simulink model "Team37_Quadcopter_Simulation"  (R2018a)
settings: Solver=ode45  StartTime=0  StopTime=10.0  FixedStep=0.005  RelTol=1e-3  EnableMultiTasking=on
model workspace (MAT data in the model file):
  Sig = Simulink.Signal
  Sig.DataType = 'auto'
  Sig.Dimensions = -1
  Sig.DimensionsMode = 'auto'
  Sig.Complexity = 'auto'
  Sig.SampleTime = -1
  Sig.SamplingMode = 'auto'
values from neighbouring files (symbols this model uses):
  IC =     [ICload.mat]
undefined symbols (not defined in the file or in its folder): DiscIntNeverNeededParam, quadModel
libraries: simulink x8
(part 1 of 2)
Description:
  | This is a configurable quadcopter simulation.
  | This Simulink model demonstates several effects intended to simulate a real-world attitude control implementation.
  | 
  | Additional quadcopter modeling and simulation materials available at:
  | github.com/dch33/Quad-Sim
  | 
  | Copyright (C) 2014 D. Hartman, K. Landis, S. Moreno, J. Kim, M. Mehrer
  | 
  | License:
  |     This program is free software: you can redistribute it and/or modify
  |     it under the terms of the GNU LESSER GENERAL PUBLIC LICENSE as published by
  |     the Free Software Foundation, either version 3 of the License, or
  |     (at your option) any later version.
  | 
  |     This program is distributed in the hope that it will be useful,
  |     but WITHOUT ANY WARRANTY; without even the implied warranty of
  |     MERCHANTABILITY or FITNESS FOR A PARTICULAR PURPOSE.  See the
  |     GNU General Public License for more details.
  | 
  |     You should have received a copy of the GNU LESSER GENERAL PUBLIC LICENSE
  |     along with this program.  If not, see <http://www.gnu.org/licenses/>.
settings Model: ModifiedComment=m203876 -- Mon Sep 02 20:57:19 2019 -- Version 1.4  Creator=David Hartman  LastModifiedBy=m203876
settings Model: ModifiedHistory=|
  | m203876 -- Mon Sep 02 20:57:19 2019 -- Version 1.4
  | 
  | davidhartman -- Fri Jun 06 23:02:32 2014 -- Version 1.3
settings SolverCC: AutoInsertRateTranBlk=on
settings DataIOCC: SaveFormat=Array  SaveState=on  SignalLogging=off
settings OptimizationCC: DefaultParameterBehavior=Inlined  LifeSpan=inf
settings DebuggingCC: UnderspecifiedInitializationDetection=Classic  MergeDetectMultiDrivingBlocksExec=none  SolverPrmCheckMsg=warning  UniqueDataStoreMsg=warning  StateNameClashWarn=warning  StrictBusMsg=WarnOnBusTreatedAsVector  SFUnexpectedBacktrackingDiag=warning  SFNoUnconditionalDefaultTransitionDiag=warning  SFExecutionAtInitializationDiag=none
settings HardwareCC: ProdBitPerPointer=32  ProdBitPerSizeT=32  ProdBitPerPtrDiffT=32  ProdLargestAtomicFloat=None  ProdIntDivRoundTo=Undefined  ProdEndianess=Unspecified  ProdWordSize=32  ProdHWDeviceType=32-bit Generic
settings ModelReferenceCC: PropagateSignalLabelsOutOfModel=off
settings CodeAppCC: StateflowObjectComments=on
settings GRTTargetCC: TargetLangStandard=C89/C90 (ANSI)  GeneratePreprocessorConditionals=Disable all
settings ConfigComp: CovMetricSettings=dw  CovHtmlReporting=on  CovSaveCumulativeToWorkspaceVar=on  CovSaveSingleToWorkspaceVar=on  CovExternalEMLEnable=off

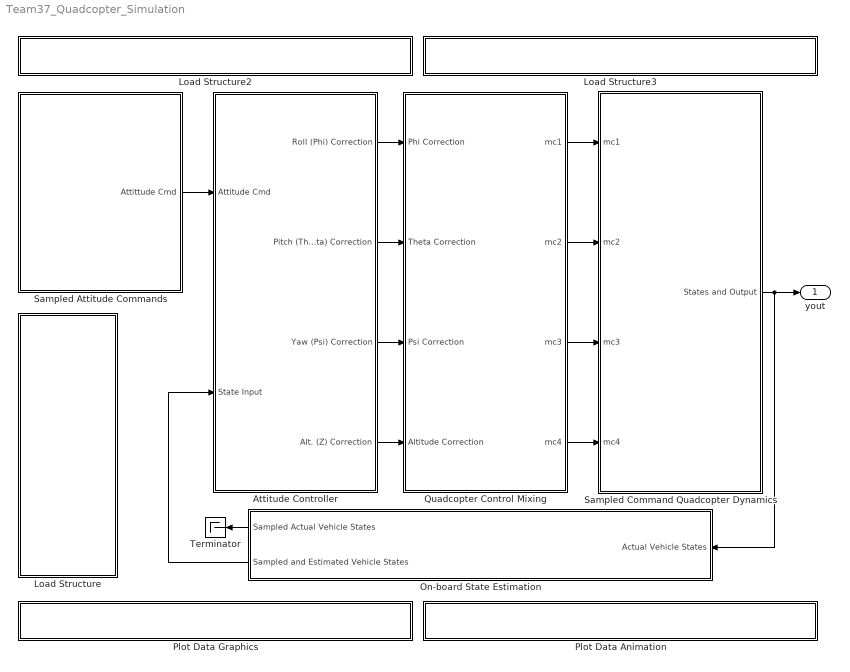
== system Team37_Quadcopter_Simulation ==
  Attitude Controller : Subsystem
  Load Structure : Subsystem
      settings: OpenFcn=|
      | uiopen('load')
      | if (exist('IC')==1 && exist('quadModel')==1)
      | set_param(bdroot, 'SimulationCommand', 'update')
      | end
      mask Display: fprintf('LOAD:\nQuadcopter\nModel Or\nInitial\nConditions');
  Load Structure2 : Subsystem
      settings: OpenFcn=|
      | if exist('GUI_Modeling') == 2,
      | run('GUI_Modeling')
      | 
      | else
      | 
      | msgbox('The desired GUI must be first added to MATLABs path.')
      | 
      | end
      mask Display: fprintf('OPEN GUI: Build New \n Model');
  Load Structure3 : Subsystem
      settings: OpenFcn=|
      | if exist('GUI_IC') == 2,
      | run('GUI_IC')
      | 
      | else
      | 
      | msgbox('The desired GUI must be first added to MATLABs path.')
      | 
      | end
      mask Display: fprintf('OPEN GUI: Create Initial \n Conditions');
  On-board State Estimation : Subsystem  mask{ControllerSampleTime=1/200, Gyro_Alpha=0.50, Accel_Alpha=0.06, EAComp=0.92}
      mask prompts: ControllerSampleTime "State sensor sampling time (s):"; Gyro_Alpha "Gyro Alpha Value:"; Accel_Alpha "Accelerometer Alpha Value:"; EAComp "Complimentary Filter Alpha (must be between 0 and 1):"
      mask Help:
      | Sampling Time: A typical value might be 0.02 to 0.002 seconds (50 Hz to 400 Hz)
      | depending on the control system and sensors used. For best simulink performance,
      | it may be necessarry to round the value a bit to achieve an integer multiple
      | relationship between motor command sampling time and state estimation sampling time.
      | See simulink documentation for more details.
      mask TypeOptions ControllerSampleTime: Rate Transition/OutPortSampleTime
      mask TypeOptions Gyro_Alpha: filterRawData()/Gyro_Alpha
      mask TypeOptions Accel_Alpha: filterRawData()/Accel_Alpha
      mask TypeOptions EAComp: State Estimation and Complimentary Mixing/EAComp
      mask Display:
      | fprintf(['Sampling Time: ' num2str(ControllerSampleTime) ' (s)']);
      | fprintf(['\n \n' num2str(1/ControllerSampleTime) ' Hz']);
  Plot Data Animation : Subsystem
      settings: OpenFcn=|
      | if exist('QuadAnim4') == 2,
      |     if exist('yout')
      | 	run('QuadAnim4');
      |     else
      |     msgbox('Simulation must be run before data can be plotted.');
      |     end
      | else                                                                          msgbox('The desired GUI must be first added to MATLABs path.')
      | end
      mask Display: fprintf('OPEN GUI: Flight Animation')
  Plot Data Graphics : Subsystem
      settings: OpenFcn=|
      | if exist('yout')
      | yout = evalin('base', 'yout');
      | tout = evalin('base', 'tout');
      | quadPlots(yout, tout)
      | else
      | msgbox('Simulation must be run before data can be plotted.')
      | end
      mask Display: fprintf('OPEN PLOT: State Data')
  Quadcopter Control Mixing : Subsystem  mask{QuantizationInterval=0.1}
      mask prompts: QuantizationInterval "Quantization interval (% throttle):"
      mask help:
      | Input desired quantization interval as Percent Throttle.
      | For example, if PWM ESC command signals are restricted to integers between
      | 1000 and 2000 us, quantization would be 0.1 % throttle.
      mask TypeOptions QuantizationInterval:
      | Quantizer1
      | /QuantizationInterval | Quantizer2
      | /QuantizationInterval | Quantizer3
      | /QuantizationInterval | Quantizer4/QuantizationInterval
      mask Display:
      | fprintf(['Quantization : ' num2str(QuantizationInterval) '%%  Throttle']);
      | modelLoaded = evalin('base','exist(''quadModel'',''var'')');
      | if (modelLoaded==1)
      |     if (evalin('base','quadModel.plusConfig'))
      |     fprintf([' \n' ' \n'  'Configuration "+"']);
      |     else if (~evalin('base','quadModel.plusConfig'))
      |         fprintf([' \n' ' \n' 'Configuration "X"']);
      |         end
      |     end
      | else
      |     fprintf([' \n' ' \n'  'Model Not Loaded']);
      | end
  Sampled Attitude Commands : Subsystem  mask{CommandSampleTime=1/200}
      mask prompts: CommandSampleTime "Attitude Command Sample Time (s):"
      mask TypeOptions CommandSampleTime: Rate Transition/OutPortSampleTime
      mask Display:
      | fprintf(['Sampling Time: ' num2str(CommandSampleTime) ' (s)\n\n\n\n\n\n\n']);
      | fprintf(['\n \n' num2str(1/CommandSampleTime) ' Hz \n\n\n\n\n\n']);
  Sampled Command Quadcopter Dynamics : Subsystem  mask{ESCSampleTime=0.02}
      mask prompts: ESCSampleTime "Motor Command Sampling Time (s):"
      mask help:
      | Input sampling rate for motor commands in seconds.
      | This rate will be applied to simulate the propagation of controller commands to the ESC's.
      | A typical value is on the order of 0.02 seconds (50 Hz).
      mask TypeOptions ESCSampleTime: Rate Transition/OutPortSampleTime
      mask Display:
      | fprintf(['Sampling Time: ' num2str(ESCSampleTime) ' (s)\n\n\n\n\n\n']);
      | fprintf(['\n \n' num2str(1/ESCSampleTime) ' Hz\n\n\n\n\n']);
  Terminator : Terminator
  yout : Outport
  wires:
  Sampled Command Quadcopter Dynamics/1(States and Output) -> yout/1, On-board State Estimation/1(Actual Vehicle States)
  Quadcopter Control Mixing/1(mc1) -> Sampled Command Quadcopter Dynamics/1(mc1)
  Quadcopter Control Mixing/2(mc2) -> Sampled Command Quadcopter Dynamics/2(mc2)
  Quadcopter Control Mixing/3(mc3) -> Sampled Command Quadcopter Dynamics/3(mc3)
  Quadcopter Control Mixing/4(mc4) -> Sampled Command Quadcopter Dynamics/4(mc4)
  Attitude Controller/1(Roll (Phi) Correction) -> Quadcopter Control Mixing/1(Phi Correction)
  Attitude Controller/3(Yaw (Psi) Correction) -> Quadcopter Control Mixing/3(Psi Correction)
  Attitude Controller/2(Pitch (Theta) Correction) -> Quadcopter Control Mixing/2(Theta Correction)
  Attitude Controller/4(Alt. (Z) Correction) -> Quadcopter Control Mixing/4(Altitude Correction)
  On-board State Estimation/2(Sampled and Estimated Vehicle States) -> Attitude Controller/2(State Input)
  On-board State Estimation/1(Sampled Actual Vehicle States) -> Terminator/1
  Sampled Attitude Commands/1(Attittude Cmd) -> Attitude Controller/1(Attitude Cmd)

== system Team37_Quadcopter_Simulation/Attitude Controller ==
  Attitude Cmd : Inport
  State Input : Inport  Port=2
  Altitude (Z) Control : Subsystem  mask{Kpz=2, Kiz=1.1, Kdz=3.0, LimitOutput=on, USat=1, LSat=-1, GOffset=(sqrt((quadModel.mass*quadModel.g)/(4*quadModel.ct))-quadModel.b)/quadModel.cr}
      mask prompts: Kpz "Kp"; Kiz "Ki"; Kdz "Kd"; LimitOutput "Integral Saturation?"; USat "Upper saturation limit:"; LSat "Lower saturation limit:"; GOffset "Gravity Feedforward"
      mask help:
      | Adjust PID controller gains through this mask interface, or "look under mask" for more detailed adjustments.
      |
      | Note: Gravity Offset will not appear on block face as a value until simulation is run if it is the result of a formula involving the quadcopter model parameters.
      mask TypeOptions Kpz: Kpz/Gain
      mask TypeOptions Kiz: Kiz/Gain
      mask TypeOptions Kdz: Kdz/Gain
      mask TypeOptions LimitOutput:
      | Discrete-Time
      | Integrator/LimitOutput
      mask TypeOptions USat:
      | Discrete-Time
      | Integrator/UpperSaturationLimit
      mask TypeOptions LSat:
      | Discrete-Time
      | Integrator/LowerSaturationLimit
      mask TypeOptions GOffset: Gravity Offset (Level Flight)/Value
      mask Display:
      | % port_label('input',1,'Z Command');
      | % port_label('input',2,'Z State');
      | % port_label('output',1,'Z Correction')
      | fprintf(['Gravity Offset = ' num2str(GOffset) '\n' ...
      |     'Kp = ' num2str(Kpz) '\n' ...
      |     'Ki = ' num2str(Kiz) '\n' ...
      |     'Kd = ' num2str(Kdz) '\n' ...
      |     'Integral Saturation: ' LimitOutput]);
      | if strcmp(LimitOutput,'on')
      |     fprintf([' \n' ' \n' ' \n' ' \n' ' \n' '\n' ...
      |         'Limits: ' num2str(USat) ' to ' num2str(LSat)]);
      | end
  Bus Selector : BusSelector  OutputSignals=Phi,P,The,Q,Psi,R,Z
  Pitch (Theta) Control : Subsystem  mask{Kpt=5.5, Kit=2.8, Kdt=3, Kdt2=3/8, LimitOutput=on, USat=10, LSat=-10}
      mask prompts: Kpt "Kp"; Kit "Ki"; Kdt "Kd"; Kdt2 "Kd2"; LimitOutput "Integral Saturation?"; USat "Upper saturation limit:"; LSat "Lower saturation limit:"
      mask help: Adjust PID controller gains through this mask interface, or "look under mask" for more detailed adjustments.
      mask TypeOptions Kpt: Kpt/Gain
      mask TypeOptions Kit: Kit/Gain
      mask TypeOptions Kdt: Kdt/Gain
      mask TypeOptions Kdt2: Kdt2/Gain
      mask TypeOptions LimitOutput:
      | Discrete-Time
      | Integrator/LimitOutput
      mask TypeOptions USat:
      | Discrete-Time
      | Integrator/UpperSaturationLimit
      mask TypeOptions LSat:
      | Discrete-Time
      | Integrator/LowerSaturationLimit
      mask Display:
      | % port_label('input',1,'Theta Command');
      | % port_label('input',2,'Theta State');
      | % port_label('input',3,'Q State');
      | % port_label('output',1,'Theta Correction');
      | fprintf(['Kp = ' num2str(Kpt) '\n' ...
      |     'Ki = ' num2str(Kit) '\n' ...
      |     'Kd = ' num2str(Kdt) '\n' ...
      |     'Kd2= ' num2str(Kdt2) '\n' ...
      |     'Integral Saturation: ' LimitOutput]);
      | if strcmp(LimitOutput,'on')
      |     fprintf([' \n' ' \n' ' \n' ' \n' '\n' '\n' ...
      |         'Limits: ' num2str(USat) ' to ' num2str(LSat)]);
      | end
  "Roll (Phi) Control " : Subsystem  mask{Kpp=3.3, Kip=0.6, Kdp=2.2, Kdp2=0.25, LimitOutput=on, USat=10, LSat=-10}
      mask prompts: Kpp "Kp"; Kip "Ki"; Kdp "Kd"; Kdp2 "Kd2"; LimitOutput "Integral Saturation:"; USat "Upper saturation limit:"; LSat "Lower saturation limit:"
      mask help:
      | Adjust PID controller gains through this mask interface, or "look under mask"
      | for more detailed adjustments.
      mask TypeOptions Kpp: Kpp/Gain
      mask TypeOptions Kip: Kip/Gain
      mask TypeOptions Kdp: Kdp/Gain
      mask TypeOptions Kdp2: Kdp2/Gain
      mask TypeOptions LimitOutput:
      | Discrete-Time
      | Integrator/LimitOutput
      mask TypeOptions USat:
      | Discrete-Time
      | Integrator/UpperSaturationLimit
      mask TypeOptions LSat:
      | Discrete-Time
      | Integrator/LowerSaturationLimit
      mask Display:
      | fprintf(['Kp = ' num2str(Kpp) '\n' ...
      |     'Ki = ' num2str(Kip) '\n' ...
      |     'Kd = ' num2str(Kdp) '\n'...
      |     'Kd2= ' num2str(Kdp2) '\n'...
      |     'Integral Saturation: ' LimitOutput]);
      | if strcmp(LimitOutput,'on')
      |     fprintf([' \n' ' \n' ' \n' ' \n' '\n' '\n' ...
      |         'Limits: ' num2str(USat) ' to ' num2str(LSat)]);
      | end
  Yaw (Psi) Control : Subsystem  mask{Kps=5, Kis=1, Kds=5, Kds2=0.3, LimitOutput=on, USat=10, LSat=-10}
      mask prompts: Kps "Kp"; Kis "Ki"; Kds "Kd"; Kds2 "Kd2"; LimitOutput "Integral Saturation?"; USat "Upper saturation limit:"; LSat "Lower saturation limit:"
      mask help: Adjust PID controller gains through this mask interface, or "look under mask" for more detailed adjustments.
      mask TypeOptions Kps: Kps/Gain
      mask TypeOptions Kis: Kit/Gain
      mask TypeOptions Kds: Kds/Gain
      mask TypeOptions Kds2: Kds2/Gain
      mask TypeOptions LimitOutput:
      | Discrete-Time
      | Integrator/LimitOutput
      mask TypeOptions USat:
      | Discrete-Time
      | Integrator/UpperSaturationLimit
      mask TypeOptions LSat:
      | Discrete-Time
      | Integrator/LowerSaturationLimit
      mask Display:
      | fprintf(['Kp = ' num2str(Kps) '\n' ...
      |     'Ki = ' num2str(Kis) '\n' ...
      |     'Kd = ' num2str(Kds) '\n' ...
      |     'Kd2 = ' num2str(Kds2) '\n' ...
      |     'Integral Saturation: ' LimitOutput]);
      | if strcmp(LimitOutput,'on')
      |     fprintf([' \n' ' \n' ' \n' ' \n' '\n' '\n' ...
      |         'Limits: ' num2str(USat) ' to ' num2str(LSat)]);
      | end
  Roll (Phi) Correction : Outport
  Pitch (Theta) Correction : Outport  Port=2
  Yaw (Psi) Correction : Outport  Port=3
  Alt. (Z) Correction : Outport  Port=4
  wires:
  "Roll (Phi) Control "/1(Phi Correction) -> Roll (Phi) Correction/1
  Bus Selector/1 -> "Roll (Phi) Control "/2(Phi State)  "<Phi>"
  State Input/1 -> Bus Selector/1
  Pitch (Theta) Control/1(Theta Correction) -> Pitch (Theta) Correction/1
  Yaw (Psi) Control/1(Psi Correction) -> Yaw (Psi) Correction/1
  Bus Selector/5 -> Yaw (Psi) Control/2(Psi State)  "<Psi>"
  Altitude (Z) Control/1(Alt. (Z) Correction) -> Alt. (Z) Correction/1
  Bus Selector/7 -> Altitude (Z) Control/2(Z State)  "<Z>"
  Attitude Cmd/1 -> Altitude (Z) Control/1(Desired Z), Yaw (Psi) Control/1(Attitude Command), Pitch (Theta) Control/1(Attitude Command), "Roll (Phi) Control "/1("Attitude Command ")
  Bus Selector/3 -> Pitch (Theta) Control/2(Theta State)  "<The>"
  Bus Selector/2 -> "Roll (Phi) Control "/3(P)  "<P>"
  Bus Selector/4 -> Pitch (Theta) Control/3(Q State)  "<Q>"
  Bus Selector/6 -> Yaw (Psi) Control/3(R State)  "<R>"

== system Team37_Quadcopter_Simulation/Load Structure ==

== system Team37_Quadcopter_Simulation/Load Structure2 ==

== system Team37_Quadcopter_Simulation/Load Structure3 ==

== system Team37_Quadcopter_Simulation/On-board State Estimation ==
  note: This block is intended to simulate the process used onboard the vehicle
      | to estimate the attitude of the quad using the MPU-6050 data and filtering algorithms.
  note: Just a pass through
  Actual Vehicle States : Inport
  B3filtRawData() : Subsystem  mask{inputGain=1/3.102185882e+03, x1x2Gain=3, y2Gain=2.7130114176, y1Gain=-2.4657422174, y0Gain=0.7501519731}
      mask prompts: inputGain "Input Gain:"; x1x2Gain "x1x2 Gain:"; y2Gain "y2 Gain:"; y1Gain "y1 Gain:"; y0Gain "y0 Gain:"
      mask TypeOptions inputGain: InputGain/Gain
      mask TypeOptions x1x2Gain: x1x2Gain/Gain
      mask TypeOptions y2Gain: y2Gain/Gain
      mask TypeOptions y1Gain: y1Gain/Gain
      mask TypeOptions y0Gain: y0Gain/Gain
  Mix Bus Output : Subsystem
  Rate Transition : RateTransition  Deterministic=off  OutPortSampleTime=ControllerSampleTime
  State Estimation and Complimentary Mixing : Subsystem  mask{EAComp=EAComp}
      mask prompts: EAComp "Complimentary Filter Alpha:"
      mask TypeOptions EAComp: Complimentary Filter/EAComp
  data scaling : Subsystem
  filterRawData() : Subsystem  mask{Gyro_Alpha=Gyro_Alpha, Accel_Alpha=Accel_Alpha}
      mask prompts: Gyro_Alpha "Gyro Alpha Value:"; Accel_Alpha "Accelerometer Alpha Value:"
      mask TypeOptions Gyro_Alpha: Gyro alpha/Gain
      mask TypeOptions Accel_Alpha: Accel alpha/Gain
  getMotion6() : Subsystem
  Sampled Actual Vehicle States : Outport
  Sampled and Estimated Vehicle States : Outport  Port=2
  wires:
  Actual Vehicle States/1 -> Rate Transition/1
  Rate Transition/1 -> getMotion6()/1(In1), Sampled Actual Vehicle States/1, Mix Bus Output/2(Sampled Actual States)
  getMotion6()/1(Out1) -> B3filtRawData()/1(In1)
  data scaling/1(Out1) -> State Estimation and Complimentary Mixing/1(In1)
  State Estimation and Complimentary Mixing/1(State Estimations) -> Mix Bus Output/1(Estimated States)
  Mix Bus Output/1(Out1) -> Sampled and Estimated Vehicle States/1
  B3filtRawData()/1(Out1) -> filterRawData()/1(In1)
  filterRawData()/1(Out1) -> data scaling/1(In1)

== system Team37_Quadcopter_Simulation/Plot Data Animation ==

== system Team37_Quadcopter_Simulation/Plot Data Graphics ==

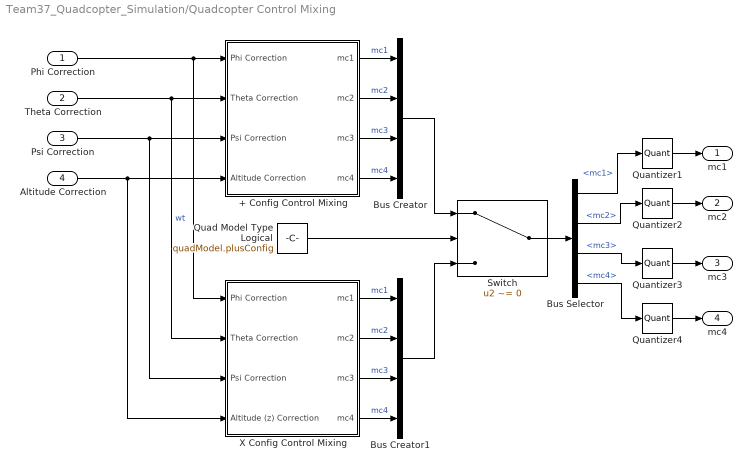
== system Team37_Quadcopter_Simulation/Quadcopter Control Mixing ==
  Phi Correction : Inport
  Theta Correction : Inport  Port=2
  Psi Correction : Inport  Port=3
  Altitude Correction : Inport  Port=4
  + Config Control Mixing : Subsystem
  Bus Creator : BusCreator  Inputs=4
  Bus Creator1 : BusCreator  Inputs=4
  Bus Selector : BusSelector  OutputSignals=mc1,mc2,mc3,mc4
  Quad Model Type Logical : Constant  Value=quadModel.plusConfig
  "Quantizer1 " : Quantizer  QuantizationInterval=QuantizationInterval
  "Quantizer2 " : Quantizer  QuantizationInterval=QuantizationInterval
  "Quantizer3 " : Quantizer  QuantizationInterval=QuantizationInterval
  Quantizer4 : Quantizer  QuantizationInterval=QuantizationInterval
  Switch : Switch  Criteria=u2 ~= 0
  X Config Control Mixing : Subsystem
  mc1 : Outport
  mc2 : Outport  Port=2
  mc3 : Outport  Port=3
  mc4 : Outport  Port=4
  wires:
  Phi Correction/1 -> X Config Control Mixing/1(Phi Correction), + Config Control Mixing/1(Phi Correction)
  Theta Correction/1 -> X Config Control Mixing/2(Theta Correction), + Config Control Mixing/2(Theta Correction)  "wt"
  Psi Correction/1 -> X Config Control Mixing/3(Psi Correction), + Config Control Mixing/3(Psi Correction)
  Altitude Correction/1 -> X Config Control Mixing/4(Altitude (z) Correction), + Config Control Mixing/4(Altitude Correction)
  + Config Control Mixing/1(mc1) -> Bus Creator/1  "mc1"
  + Config Control Mixing/2(mc2) -> Bus Creator/2  "mc2"
  + Config Control Mixing/3(mc3) -> Bus Creator/3  "mc3"
  + Config Control Mixing/4(mc4) -> Bus Creator/4  "mc4"
  Bus Creator/1 -> Switch/1
  X Config Control Mixing/1(mc1) -> Bus Creator1/1  "mc1"
  X Config Control Mixing/2(mc2) -> Bus Creator1/2  "mc2"
  X Config Control Mixing/3(mc3) -> Bus Creator1/3  "mc3"
  X Config Control Mixing/4(mc4) -> Bus Creator1/4  "mc4"
  Bus Creator1/1 -> Switch/3
  Bus Selector/1 -> "Quantizer1 "/1  "<mc1>"
  Bus Selector/2 -> "Quantizer2 "/1  "<mc2>"
  Bus Selector/3 -> "Quantizer3 "/1  "<mc3>"
  Bus Selector/4 -> Quantizer4/1  "<mc4>"
  Quad Model Type Logical/1 -> Switch/2
  Switch/1 -> Bus Selector/1
  "Quantizer1 "/1 -> mc1/1
  "Quantizer2 "/1 -> mc2/1
  "Quantizer3 "/1 -> mc3/1
  Quantizer4/1 -> mc4/1

== system Team37_Quadcopter_Simulation/Sampled Attitude Commands ==
  Bus Creator : BusCreator  Inputs=4
  Rate Transition : RateTransition  OutPortSampleTime=CommandSampleTime
  Step : Step  Time=2.0  After=0  SampleTime=0
  Step1 : Step  Time=0  After=10*pi/180  SampleTime=0
  Step2 : Step  Time=0  After=0  SampleTime=0
  Step3 : Step  Time=7.5  Before=10*0.3048  After=10*0.3048  SampleTime=0
  Attittude Cmd : Outport
  tag scope: A=global
  wires:
  Step/1 -> Bus Creator/1  "Phi_cmd"
  Step1/1 -> Bus Creator/2  "The_cmd"
  Step2/1 -> Bus Creator/3  "Psi_cmd"
  Step3/1 -> Bus Creator/4  "Alt_cmd"
  Bus Creator/1 -> Rate Transition/1
  Rate Transition/1 -> [A], Attittude Cmd/1  "Attitude_Cmd"

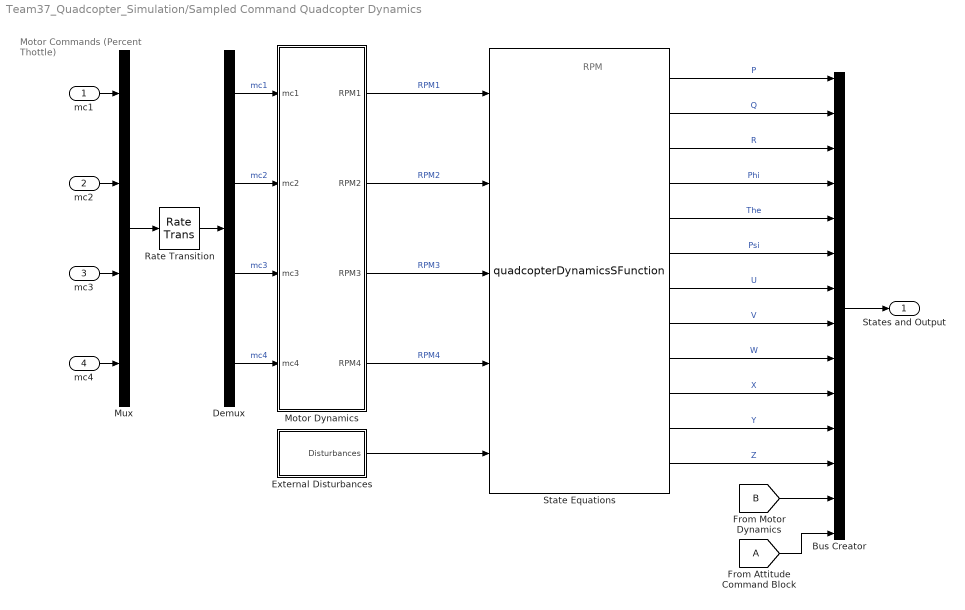
== system Team37_Quadcopter_Simulation/Sampled Command Quadcopter Dynamics ==
  note: RPM
  note: Motor Commands
      | (Percent Thottle)
  mc1 : Inport
  mc2 : Inport  Port=2
  mc3 : Inport  Port=3
  mc4 : Inport  Port=4
  Bus Creator : BusCreator  Inputs='P','Q','R','Phi','The','Psi','U','V','W','X','Y','Z','mc and RPM','Attitude_Cmd'
  Demux : Demux
  External Disturbances : Subsystem
  Motor Dynamics : Subsystem
  Mux : Mux
  Rate Transition : RateTransition  Deterministic=off  OutPortSampleTime=ESCSampleTime
  State Equations : M-S-Function  FunctionName=quadcopterDynamicsSFunction  Parameters=quadModel, IC
      mask Display:
      | port_label('input', 1, 'RPM1')
      | port_label('input', 2, 'RPM2')
      | port_label('input', 3, 'RPM3')
      | port_label('input', 4, 'RPM4')
      | port_label('input', 5, 'Disturbances')
      | port_label('output', 1, 'P')
      | port_label('output', 2, 'Q')
      | port_label('output', 3, 'R')
      | port_label('output', 4, 'Phi')
      | port_label('output', 5, 'The')
      | port_label('output', 6, 'Psi')
      | port_label('output', 7, 'U')
      | port_label('output', 8, 'V')
      | port_label('output', 9, 'W')
      | port_label('output', 10, 'X')
      | port_label('output', 11, 'Y')
      | port_label('output', 12, 'Z')
  States and Output : Outport
  wires:
  mc1/1 -> Mux/1
  mc2/1 -> Mux/2
  mc3/1 -> Mux/3
  mc4/1 -> Mux/4
  State Equations/1 -> Bus Creator/1  "P"
  State Equations/2 -> Bus Creator/2  "Q"
  State Equations/3 -> Bus Creator/3  "R"
  State Equations/4 -> Bus Creator/4  "Phi"
  State Equations/5 -> Bus Creator/5  "The"
  State Equations/6 -> Bus Creator/6  "Psi"
  State Equations/7 -> Bus Creator/7  "U"
  State Equations/8 -> Bus Creator/8  "V"
  State Equations/9 -> Bus Creator/9  "W"
  State Equations/10 -> Bus Creator/10  "X"
  State Equations/11 -> Bus Creator/11  "Y"
  State Equations/12 -> Bus Creator/12  "Z"
  Bus Creator/1 -> States and Output/1
  Motor Dynamics/1(RPM1) -> State Equations/1  "RPM1"
  Motor Dynamics/2(RPM2) -> State Equations/2  "RPM2"
  Motor Dynamics/3(RPM3) -> State Equations/3  "RPM3"
  Motor Dynamics/4(RPM4) -> State Equations/4  "RPM4"
  Demux/1 -> Motor Dynamics/1(mc1)  "mc1"
  Demux/4 -> Motor Dynamics/4(mc4)  "mc4"
  Demux/3 -> Motor Dynamics/3(mc3)  "mc3"
  Demux/2 -> Motor Dynamics/2(mc2)  "mc2"
  Mux/1 -> Rate Transition/1
  Rate Transition/1 -> Demux/1
  External Disturbances/1("Disturbances ") -> State Equations/5
  [A] -> Bus Creator/14
  [B] -> Bus Creator/13

== system Team37_Quadcopter_Simulation/Attitude Controller/Altitude (Z) Control ==
  note: ez
  Desired Z : Inport
  Z State : Inport  Port=2
  Bus Selector : BusSelector  OutputSignals=Alt_cmd
  Derivative IC fixer : Subsystem
  Discrete Derivative : simulink/Discrete/Discrete Derivative  gainval=1.0  ICPrevScaledInput=0.0  InputProcessing=Inherited  OutMin=[]  OutMax=[]  OutDataType=fixdt(1, 16)  OutScaling=2^-10  DoSatur=off
  Discrete-Time Integrator : DiscreteIntegrator  IntegratorMethod=Integration: Backward Euler  SampleTime=-1  LimitOutput=on  UpperSaturationLimit=USat  LowerSaturationLimit=LSat  ICPrevOutput=DiscIntNeverNeededParam  ICPrevScaledInput=DiscIntNeverNeededParam
  Gravity Offset (Level Flight) : Constant  Value=GOffset
  Initial Derivative : Constant  Value=0
  Kdz : Gain  Gain=Kdz
  Kiz : Gain  Gain=Kiz
  Kpz : Gain  Gain=Kpz
  Sum : Sum  Inputs=|+-
  Sum2 : Sum  Inputs=+++-
  Alt. (Z) Correction : Outport
  wires:
  Gravity Offset (Level Flight)/1 -> Sum2/1
  Desired Z/1 -> Bus Selector/1
  Z State/1 -> Discrete Derivative/1, Sum/2
  Sum2/1 -> Alt. (Z) Correction/1
  Kpz/1 -> Sum2/2  "P Corr"
  Sum/1 -> Discrete-Time Integrator/1, Kpz/1  "Error"
  Kiz/1 -> Sum2/3  "I Corr"
  Kdz/1 -> Sum2/4  "D Corr"
  Discrete-Time Integrator/1 -> Kiz/1
  Discrete Derivative/1 -> Derivative IC fixer/2(Normal Output)
  Bus Selector/1 -> Sum/1  "<Alt_cmd>"
  Initial Derivative/1 -> Derivative IC fixer/1(FilterStart)
  Derivative IC fixer/1(Out1) -> Kdz/1

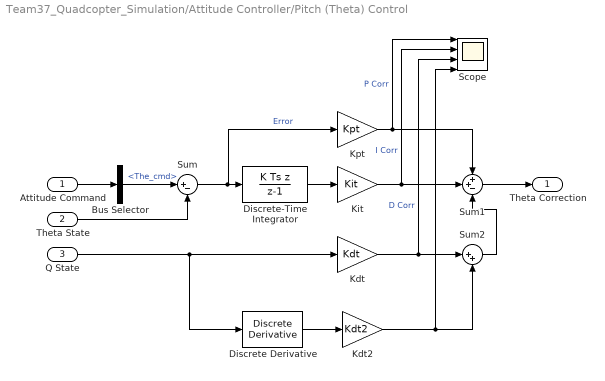
== system Team37_Quadcopter_Simulation/Attitude Controller/Pitch (Theta) Control ==
  Attitude Command : Inport
  Theta State : Inport  Port=2
  Q State : Inport  Port=3
  Bus Selector : BusSelector  OutputSignals=The_cmd
  Discrete Derivative : simulink/Discrete/Discrete Derivative  gainval=1.0  ICPrevScaledInput=0.0  InputProcessing=Inherited  OutMin=[]  OutMax=[]  OutDataType=fixdt(1, 16)  OutScaling=2^-10  DoSatur=off
  Discrete-Time Integrator : DiscreteIntegrator  IntegratorMethod=Integration: Backward Euler  SampleTime=-1  LimitOutput=on  UpperSaturationLimit=USat  LowerSaturationLimit=LSat  ICPrevOutput=DiscIntNeverNeededParam  ICPrevScaledInput=DiscIntNeverNeededParam
  Kdt : Gain  Gain=Kdt
  Kdt2 : Gain  Gain=Kdt2
  Kit : Gain  Gain=Kit
  Kpt : Gain  Gain=Kpt
  Scope : Scope  NumInputPorts=4
  Sum : Sum  Inputs=|+-
  Sum1 : Sum  Inputs=++-
  Sum2 : Sum  Inputs=|++
  Theta Correction : Outport
  wires:
  Sum/1 -> Discrete-Time Integrator/1, Kpt/1  "Error"
  Attitude Command/1 -> Bus Selector/1
  Theta State/1 -> Sum/2
  Discrete-Time Integrator/1 -> Kit/1
  Bus Selector/1 -> Sum/1  "<The_cmd>"
  Q State/1 -> Discrete Derivative/1, Kdt/1
  Kpt/1 -> Scope/1, Sum1/1  "P Corr"
  Kit/1 -> Scope/2, Sum1/2  "I Corr"
  Sum1/1 -> Theta Correction/1
  Discrete Derivative/1 -> Kdt2/1
  Sum2/1 -> Sum1/3
  Kdt2/1 -> Sum2/2, Scope/4
  Kdt/1 -> Sum2/1, Scope/3  "D Corr"

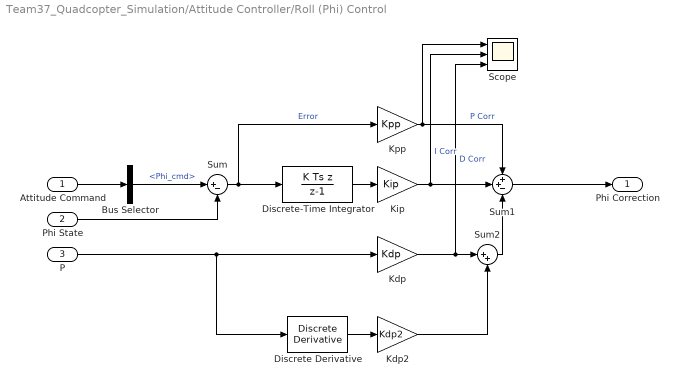
== system Team37_Quadcopter_Simulation/Attitude Controller/Roll (Phi) Control  ==
  "Attitude Command " : Inport
  Phi State : Inport  Port=2
  P : Inport  Port=3
  Bus Selector : BusSelector  OutputSignals=Phi_cmd
  Discrete Derivative : simulink/Discrete/Discrete Derivative  gainval=1.0  ICPrevScaledInput=0.0  InputProcessing=Inherited  OutMin=[]  OutMax=[]  OutDataType=fixdt(1, 16)  OutScaling=2^-10  DoSatur=off
  Discrete-Time Integrator : DiscreteIntegrator  IntegratorMethod=Integration: Backward Euler  SampleTime=-1  LimitOutput=on  UpperSaturationLimit=USat  LowerSaturationLimit=LSat  ICPrevOutput=DiscIntNeverNeededParam  ICPrevScaledInput=DiscIntNeverNeededParam
  Kdp : Gain  Gain=Kdp
  Kdp2 : Gain  Gain=Kdp2
  Kip : Gain  Gain=Kip
  Kpp : Gain  Gain=Kpp
  Scope : Scope  NumInputPorts=3
  Sum : Sum  Inputs=|+-
  Sum1 : Sum  Inputs=++-
  Sum2 : Sum  Inputs=|++
  Phi Correction : Outport
  wires:
  Sum/1 -> Discrete-Time Integrator/1, Kpp/1  "Error"
  Phi State/1 -> Sum/2
  Sum1/1 -> Phi Correction/1
  Kpp/1 -> Scope/1, Sum1/1  "P Corr"
  Kdp/1 -> Sum2/1, Scope/3  "D Corr"
  Kip/1 -> Scope/2, Sum1/2  "I Corr"
  Discrete-Time Integrator/1 -> Kip/1
  "Attitude Command "/1 -> Bus Selector/1
  Bus Selector/1 -> Sum/1  "<Phi_cmd>"
  P/1 -> Discrete Derivative/1, Kdp/1
  Discrete Derivative/1 -> Kdp2/1
  Kdp2/1 -> Sum2/2
  Sum2/1 -> Sum1/3

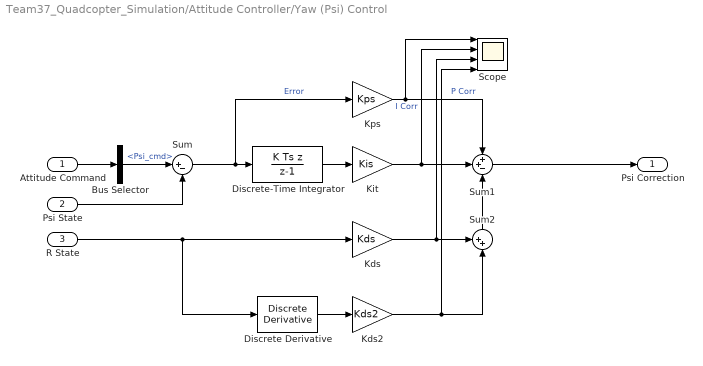
== system Team37_Quadcopter_Simulation/Attitude Controller/Yaw (Psi) Control ==
  Attitude Command : Inport
  Psi State : Inport  Port=2
  R State : Inport  Port=3
  Bus Selector : BusSelector  OutputSignals=Psi_cmd
  Discrete Derivative : simulink/Discrete/Discrete Derivative  gainval=1.0  ICPrevScaledInput=0.0  InputProcessing=Inherited  OutMin=[]  OutMax=[]  OutDataType=fixdt(1, 16)  OutScaling=2^-10  DoSatur=off
  Discrete-Time Integrator : DiscreteIntegrator  IntegratorMethod=Integration: Backward Euler  SampleTime=-1  LimitOutput=on  UpperSaturationLimit=USat  LowerSaturationLimit=LSat  ICPrevOutput=DiscIntNeverNeededParam  ICPrevScaledInput=DiscIntNeverNeededParam
  Kds : Gain  Gain=Kds
  Kds2 : Gain  Gain=Kds2
  Kit : Gain  Gain=Kis
  Kps : Gain  Gain=Kps
  Scope : Scope  NumInputPorts=4
  Sum : Sum  Inputs=|+-
  Sum1 : Sum  Inputs=++-
  Sum2 : Sum  Inputs=++|
  Psi Correction : Outport
  wires:
  Sum/1 -> Discrete-Time Integrator/1, Kps/1  "Error"
  Attitude Command/1 -> Bus Selector/1
  Sum1/1 -> Psi Correction/1
  Psi State/1 -> Sum/2
  Kps/1 -> Scope/1, Sum1/1  "P Corr"
  Kds/1 -> Sum2/1, Scope/3
  Kit/1 -> Scope/2, Sum1/2  "I Corr"
  Discrete-Time Integrator/1 -> Kit/1
  Bus Selector/1 -> Sum/1  "<Psi_cmd>"
  R State/1 -> Discrete Derivative/1, Kds/1
  Discrete Derivative/1 -> Kds2/1
  Kds2/1 -> Scope/4, Sum2/2
  Sum2/1 -> Sum1/3

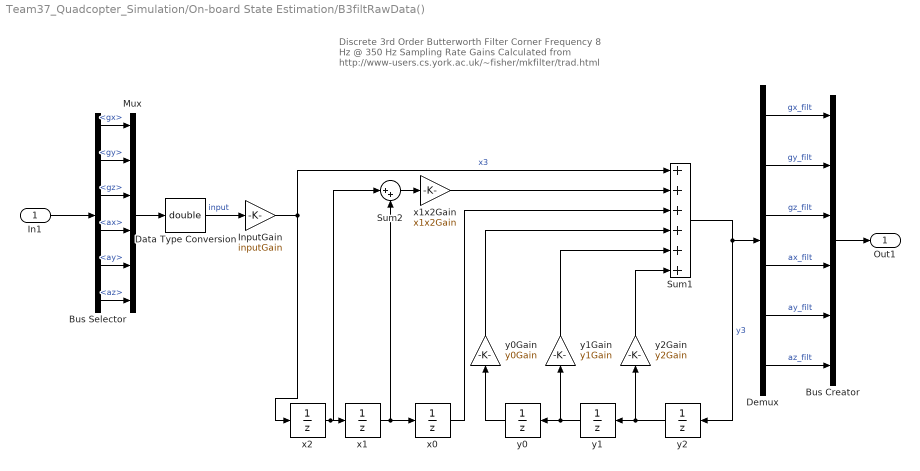
== system Team37_Quadcopter_Simulation/On-board State Estimation/B3filtRawData() ==
  note: Discrete
      | 3rd Order Butterworth Filter
      | Corner Frequency 8 Hz @ 350 Hz Sampling Rate
      | Gains Calculated from
      | http://www-users.cs.york.ac.uk/~fisher/mkfilter/trad.html
  In1 : Inport
  Bus Creator : BusCreator  Inputs=6
  Bus Selector : BusSelector  OutputSignals=gx,gy,gz,ax,ay,az
  Data Type Conversion : DataTypeConversion  OutDataTypeStr=double  RndMeth=Nearest
  Demux : Demux  Outputs=6
  InputGain : Gain  Gain=inputGain
  Mux : Mux  Inputs=6
  Sum1 : Sum  Inputs=++++++
  Sum2 : Sum  Inputs=|++
  x0 : UnitDelay  SampleTime=-1
  x1 : UnitDelay  SampleTime=-1
  x1x2Gain : Gain  Gain=x1x2Gain
  x2 : UnitDelay  SampleTime=-1
  y0 : UnitDelay  SampleTime=-1
  y0Gain : Gain  Gain=y0Gain
  y1 : UnitDelay  SampleTime=-1
  y1Gain : Gain  Gain=y1Gain
  y2 : UnitDelay  SampleTime=-1
  y2Gain : Gain  Gain=y2Gain
  Out1 : Outport
  wires:
  Sum1/1 -> Demux/1, y2/1  "y3"
  In1/1 -> Bus Selector/1
  Bus Selector/1 -> Mux/1  "<gx>"
  Bus Selector/2 -> Mux/2  "<gy>"
  Bus Selector/3 -> Mux/3  "<gz>"
  Mux/1 -> Data Type Conversion/1
  Demux/1 -> Bus Creator/1  "gx_filt"
  Demux/2 -> Bus Creator/2  "gy_filt"
  Demux/3 -> Bus Creator/3  "gz_filt"
  Bus Creator/1 -> Out1/1
  Data Type Conversion/1 -> InputGain/1  "input"
  Bus Selector/4 -> Mux/4  "<ax>"
  Bus Selector/5 -> Mux/5  "<ay>"
  Bus Selector/6 -> Mux/6  "<az>"
  Demux/4 -> Bus Creator/4  "ax_filt"
  Demux/5 -> Bus Creator/5  "ay_filt"
  Demux/6 -> Bus Creator/6  "az_filt"
  y2/1 -> y2Gain/1, y1/1
  y1/1 -> y1Gain/1, y0/1
  InputGain/1 -> x2/1, Sum1/1  "x3"
  x2/1 -> Sum2/1, x1/1
  x1/1 -> Sum2/2, x0/1
  Sum2/1 -> x1x2Gain/1
  x1x2Gain/1 -> Sum1/2
  y0Gain/1 -> Sum1/4
  y0/1 -> y0Gain/1
  y1Gain/1 -> Sum1/5
  y2Gain/1 -> Sum1/6
  x0/1 -> Sum1/3

== system Team37_Quadcopter_Simulation/On-board State Estimation/Mix Bus Output ==
  note: These states are sampled actual values
      | not used by the stability controller
  note: These are the estimated states
  Estimated States : Inport
  Sampled Actual States : Inport  Port=2
  Bus Creator : BusCreator  Inputs=12
  Bus Selector1 : BusSelector  OutputSignals=U,V,W,X,Y,Z
  Bus Selector2 : BusSelector  OutputSignals=P,Q,R,Phi,The,Psi
  Debug Scopes For Comparing Actual Versus Estimated Outputs This illustrates some of the effects from filtering : Subsystem
  Out1 : Outport
  wires:
  Bus Selector2/2 -> Bus Creator/2  "<Q>"
  Bus Selector2/3 -> Bus Creator/3  "<R>"
  Bus Selector2/1 -> Bus Creator/1  "<P>"
  Bus Selector2/5 -> Bus Creator/5  "<The>"
  Bus Selector1/5 -> Bus Creator/11  "<Y>"
  Bus Selector1/4 -> Bus Creator/10  "<X>"
  Bus Selector1/1 -> Bus Creator/7  "<U>"
  Estimated States/1 -> Debug Scopes For Comparing Actual Versus Estimated Outputs This illustrates some of the effects from filtering/1(Estimated), Bus Selector2/1
  Bus Selector2/4 -> Bus Creator/4  "<Phi>"
  Bus Selector1/2 -> Bus Creator/8  "<V>"
  Bus Selector1/6 -> Bus Creator/12  "<Z>"
  Bus Creator/1 -> Out1/1
  Sampled Actual States/1 -> Debug Scopes For Comparing Actual Versus Estimated Outputs This illustrates some of the effects from filtering/2(Actual), Bus Selector1/1
  Bus Selector1/3 -> Bus Creator/9  "<W>"
  Bus Selector2/6 -> Bus Creator/6  "<Psi>"

== system Team37_Quadcopter_Simulation/On-board State Estimation/State Estimation and Complimentary Mixing ==
  note: The specific state estimation procedure employed in these bocks is
      | to be considered experimental (like everything else in this simulation).
      | While functional within the context of our application, this is not to be taken
      | as a "correct" method for state estimation or gyro/accelerometer data combination.
  note: Note:
      | x_gyro is taken as P,
      | y_gyro as Q,
      | z_gyro ad R.
  In1 : Inport
  Bus Creator : BusCreator  Inputs=6
  Bus Selector : BusSelector  OutputSignals=P,Q,R,x_acc,y_acc,z_acc
  Complimentary Filter : Subsystem  mask{EAComp=EAComp}
      mask prompts: EAComp "Complimentary Filter Alpha:"
      mask TypeOptions EAComp: EAComp1/Gain
  Subsystem : Subsystem
  Subsystem1 : Subsystem
  State Estimations : Outport
  wires:
  In1/1 -> Bus Selector/1
  Bus Selector/1 -> Bus Creator/4, Subsystem/3(P)  "<P>"
  Bus Selector/3 -> Bus Creator/6, Subsystem/5(R)  "<R>"
  Bus Selector/2 -> Bus Creator/5, Subsystem/4(Q)  "<Q>"
  Subsystem/2(thetaDot_gyro) -> Complimentary Filter/2(theDot_gyro)  "thateDot_gyro"
  Subsystem/3(psiDot_gyro) -> Complimentary Filter/3(psiDot_gyro)  "psiDot_gyro"
  Subsystem/1(phiDot_gyro) -> Complimentary Filter/1(phiDot_gyro)  "phiDot_gyro"
  Complimentary Filter/1(phi_est) -> Bus Creator/1, Subsystem/1(Phi)  "Phi"
  Complimentary Filter/2(theta_est) -> Bus Creator/2, Subsystem/2(Theta)  "The"
  Complimentary Filter/3(psi_est) -> Bus Creator/3  "Psi"
  Subsystem1/2(phi_acc) -> Complimentary Filter/5(phiDot_acc)  "phi_acc"
  Subsystem1/1(theta_acc) -> Complimentary Filter/4(the_acc)  "theta_acc"
  Bus Selector/4 -> Subsystem1/1(x_acc)  "<x_acc>"
  Bus Selector/5 -> Subsystem1/2(y_acc)  "<y_acc>"
  Bus Selector/6 -> Subsystem1/3(z_acc)  "<z_acc>"
  Bus Creator/1 -> State Estimations/1

== system Team37_Quadcopter_Simulation/On-board State Estimation/data scaling ==
  note: For simulation, no
      | offset value is calculated.
  In1 : Inport
  Bus Creator : BusCreator  Inputs=6
  Bus Selector : BusSelector  OutputSignals=gx_filt,gy_filt,gz_filt,ax_filt,ay_filt,az_filt
  Demux : Demux  Outputs=3
  Demux1 : Demux  Outputs=3
  Gain : Gain  Gain=pi/(180*131)
  Gain1 : Gain  Gain=9.81*16384
  Mux1 : Mux  Inputs=3
  Mux2 : Mux  Inputs=3
  Out1 : Outport
  wires:
  In1/1 -> Bus Selector/1
  Bus Selector/1 -> Mux1/1  "<gx_filt>"
  Bus Selector/2 -> Mux1/2  "<gy_filt>"
  Bus Selector/3 -> Mux1/3  "<gz_filt>"
  Bus Selector/4 -> Mux2/1  "<ax_filt>"
  Bus Selector/5 -> Mux2/2  "<ay_filt>"
  Bus Selector/6 -> Mux2/3  "<az_filt>"
  Mux2/1 -> Gain1/1
  Mux1/1 -> Gain/1
  Gain1/1 -> Demux1/1
  Gain/1 -> Demux/1
  Demux/1 -> Bus Creator/1  "P"
  Demux/2 -> Bus Creator/2  "Q"
  Demux/3 -> Bus Creator/3  "R"
  Demux1/1 -> Bus Creator/4  "x_acc"
  Demux1/2 -> Bus Creator/5  "y_acc"
  Demux1/3 -> Bus Creator/6  "z_acc"
  Bus Creator/1 -> Out1/1

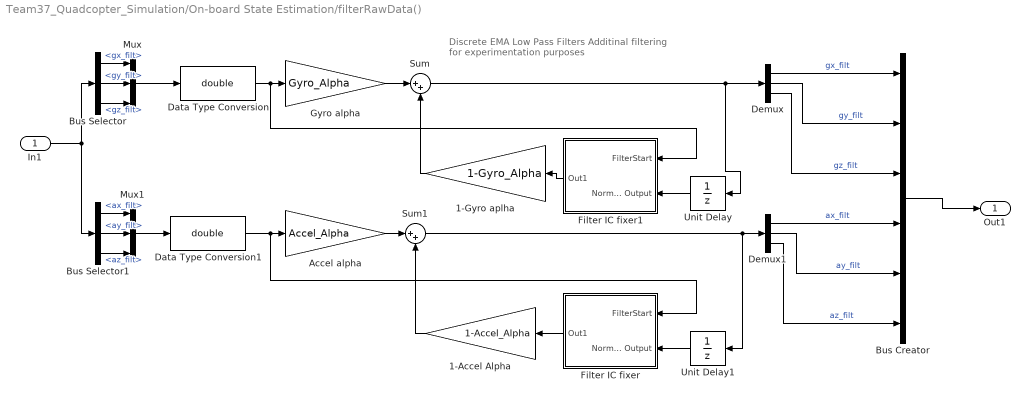
== system Team37_Quadcopter_Simulation/On-board State Estimation/filterRawData() ==
  note: Discrete EMA
      | Low Pass Filters
      | Additinal filtering for experimentation purposes
  In1 : Inport
  1-Accel Alpha : Gain  Gain=1-Accel_Alpha
  1-Gyro aplha : Gain  Gain=1-Gyro_Alpha
  Accel alpha : Gain  Gain=Accel_Alpha
  Bus Creator : BusCreator  Inputs=6
  Bus Selector : BusSelector  OutputSignals=gx_filt,gy_filt,gz_filt
  Bus Selector1 : BusSelector  OutputSignals=ax_filt,ay_filt,az_filt
  Data Type Conversion : DataTypeConversion  OutDataTypeStr=double  RndMeth=Nearest
  Data Type Conversion1 : DataTypeConversion  OutDataTypeStr=double  RndMeth=Nearest
  Demux : Demux  Outputs=3
  Demux1 : Demux  Outputs=3
  Filter IC fixer : Subsystem
  Filter IC fixer1 : Subsystem
  Gyro alpha : Gain  Gain=Gyro_Alpha
  Mux : Mux  Inputs=3
  Mux1 : Mux  Inputs=3
  Sum : Sum  Inputs=|++
  Sum1 : Sum  Inputs=|++
  Unit Delay : UnitDelay  SampleTime=-1
  Unit Delay1 : UnitDelay  SampleTime=-1
  Out1 : Outport
  wires:
  Gyro alpha/1 -> Sum/1
  Sum/1 -> Demux/1, Unit Delay/1
  In1/1 -> Bus Selector1/1, Bus Selector/1
  Accel alpha/1 -> Sum1/1
  1-Gyro aplha/1 -> Sum/2
  1-Accel Alpha/1 -> Sum1/2
  Unit Delay1/1 -> Filter IC fixer/2(Normal Output)
  Filter IC fixer/1(Out1) -> 1-Accel Alpha/1
  Unit Delay/1 -> Filter IC fixer1/2(Normal Output)
  Filter IC fixer1/1(Out1) -> 1-Gyro aplha/1
  Bus Selector/1 -> Mux/1  "<gx_filt>"
  Bus Selector/2 -> Mux/2  "<gy_filt>"
  Bus Selector/3 -> Mux/3  "<gz_filt>"
  Mux/1 -> Data Type Conversion/1
  Demux/1 -> Bus Creator/1  "gx_filt"
  Demux/2 -> Bus Creator/2  "gy_filt"
  Demux/3 -> Bus Creator/3  "gz_filt"
  Bus Creator/1 -> Out1/1
  Mux1/1 -> Data Type Conversion1/1
  Bus Selector1/1 -> Mux1/1  "<ax_filt>"
  Bus Selector1/2 -> Mux1/2  "<ay_filt>"
  Bus Selector1/3 -> Mux1/3  "<az_filt>"
  Sum1/1 -> Unit Delay1/1, Demux1/1
  Demux1/1 -> Bus Creator/4  "ax_filt"
  Demux1/2 -> Bus Creator/5  "ay_filt"
  Demux1/3 -> Bus Creator/6  "az_filt"
  Data Type Conversion/1 -> Filter IC fixer1/1(FilterStart), Gyro alpha/1
  Data Type Conversion1/1 -> Filter IC fixer/1(FilterStart), Accel alpha/1

== system Team37_Quadcopter_Simulation/On-board State Estimation/getMotion6() ==
  note: Simulate getMotion()
  note: Get std measurement from sensor
      | connect to front mask
  In1 : Inport
  Accelerometer : Subsystem
  Bus Creator : BusCreator  Inputs=6
  Bus Selector : BusSelector  OutputSignals=P,Q,R,Phi,The
  Gyro signals : Subsystem
  Out1 : Outport
  wires:
  Bus Selector/2 -> Gyro signals/2(Q)  "<Q>"
  Bus Selector/1 -> Gyro signals/1(P)  "<P>"
  Gyro signals/2(gy) -> Bus Creator/2  "gy"
  Accelerometer/1(ax) -> Bus Creator/4  "ax"
  Bus Selector/5 -> Accelerometer/2(Theta)  "<The>"
  Bus Selector/4 -> Accelerometer/1(Phi)  "<Phi>"
  Bus Selector/3 -> Gyro signals/3(R)  "<R>"
  Gyro signals/1(gx) -> Bus Creator/1  "gx"
  In1/1 -> Bus Selector/1
  Gyro signals/3(gz) -> Bus Creator/3  "gz"
  Accelerometer/2(ay) -> Bus Creator/5  "ay"
  Accelerometer/3(az) -> Bus Creator/6  "az"
  Bus Creator/1 -> Out1/1

== system Team37_Quadcopter_Simulation/Quadcopter Control Mixing/+ Config Control Mixing ==
  note: mc2 = Alt_cor + Psi_cor + Phi_cor
  note: + (plus) Quad Configuration Control Mixing
  note: mc4 = Alt_cor + Psi_cor - Phi_cor
  note: mc3 = Alt_cor - Psi_cor + The_cor
  note: mc1 = Alt_cor -Psi_cor - The_cor
  Phi Correction : Inport
  Theta Correction : Inport  Port=2
  Psi Correction : Inport  Port=3
  Altitude Correction : Inport  Port=4
  Sum1 : Sum  Inputs=|+-
  Sum11 : Sum  Inputs=-+|
  Sum2 : Sum  Inputs=|+-
  Sum3 : Sum  Inputs=++|
  Sum4 : Sum  Inputs=++|
  Sum8 : Sum  Inputs=|++
  mc1 : Outport
  mc2 : Outport  Port=2
  mc3 : Outport  Port=3
  mc4 : Outport  Port=4
  wires:
  Theta Correction/1 -> Sum1/2, Sum3/1
  Altitude Correction/1 -> Sum2/1, Sum4/2
  Sum2/1 -> Sum3/2, Sum1/1
  Psi Correction/1 -> Sum4/1, Sum2/2
  Sum4/1 -> Sum11/2, Sum8/1
  Phi Correction/1 -> Sum8/2, Sum11/1
  Sum1/1 -> mc1/1
  Sum3/1 -> mc3/1
  Sum8/1 -> mc2/1
  Sum11/1 -> mc4/1

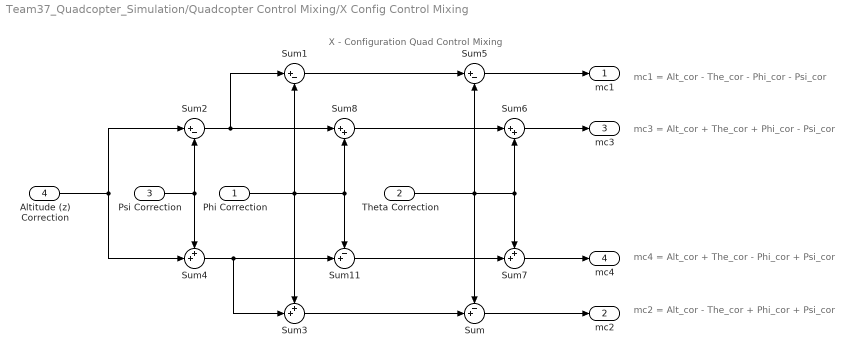
== system Team37_Quadcopter_Simulation/Quadcopter Control Mixing/X Config Control Mixing ==
  note: mc1 = Alt_cor - The_cor - Phi_cor - Psi_cor
  note: X - Configuration Quad Control Mixing
  note: mc3 = Alt_cor + The_cor + Phi_cor - Psi_cor
  note: mc2 = Alt_cor - The_cor + Phi_cor + Psi_cor
  note: mc4 = Alt_cor + The_cor - Phi_cor + Psi_cor
  Phi Correction : Inport
  Theta Correction : Inport  Port=2
  Psi Correction : Inport  Port=3
  Altitude (z) Correction : Inport  Port=4
  Sum : Sum  Inputs=-+|
  Sum1 : Sum  Inputs=|+-
  Sum11 : Sum  Inputs=-+|
  Sum2 : Sum  Inputs=|+-
  Sum3 : Sum  Inputs=++|
  Sum4 : Sum  Inputs=++|
  Sum5 : Sum  Inputs=|+-
  Sum6 : Sum  Inputs=|++
  Sum7 : Sum  Inputs=++|
  Sum8 : Sum  Inputs=|++
  mc1 : Outport
  mc2 : Outport  Port=2
  mc3 : Outport  Port=3
  mc4 : Outport  Port=4
  wires:
  Sum2/1 -> Sum8/1, Sum1/1
  Psi Correction/1 -> Sum4/1, Sum2/2
  Phi Correction/1 -> Sum3/1, Sum1/2, Sum8/2, Sum11/1
  Sum4/1 -> Sum3/2, Sum11/2
  Sum3/1 -> Sum/2
  Theta Correction/1 -> Sum7/1, Sum6/2, Sum5/2, Sum/1
  Sum1/1 -> Sum5/1
  Sum8/1 -> Sum6/1
  Sum11/1 -> Sum7/2
  Sum5/1 -> mc1/1
  Sum6/1 -> mc3/1
  Sum7/1 -> mc4/1
  Altitude (z) Correction/1 -> Sum2/1, Sum4/2
  Sum/1 -> mc2/1

== system Team37_Quadcopter_Simulation/Sampled Command Quadcopter Dynamics/External Disturbances ==
  note: Note: Torques are in units of N*m, Forces in N
      | Torques are applied to the BODY coordinate system.
      | Forces are applied from the WORLD coordinate system!
      | This can be changed by adjusting the equations within the S-function.
  Bus Creator : BusCreator  Inputs=6
  Bus to Vector : BusToVector
  Constant{2..6} (5 alike) : Constant  Value=0
  Step : Step  After=0  SampleTime=0
  "Disturbances " : Outport
  wires:
  Bus to Vector/1 -> "Disturbances "/1
  Bus Creator/1 -> Bus to Vector/1
  Constant6/1 -> Bus Creator/1  "Tau_bx-axis"
  Step/1 -> Bus Creator/2  "Tau_by-axis"
  Constant2/1 -> Bus Creator/3  "Tau_bz-axis"
  Constant3/1 -> Bus Creator/4  "Force_x-axis"
  Constant4/1 -> Bus Creator/5  "Force_y-axis"
  Constant5/1 -> Bus Creator/6  "Force_z-axis"

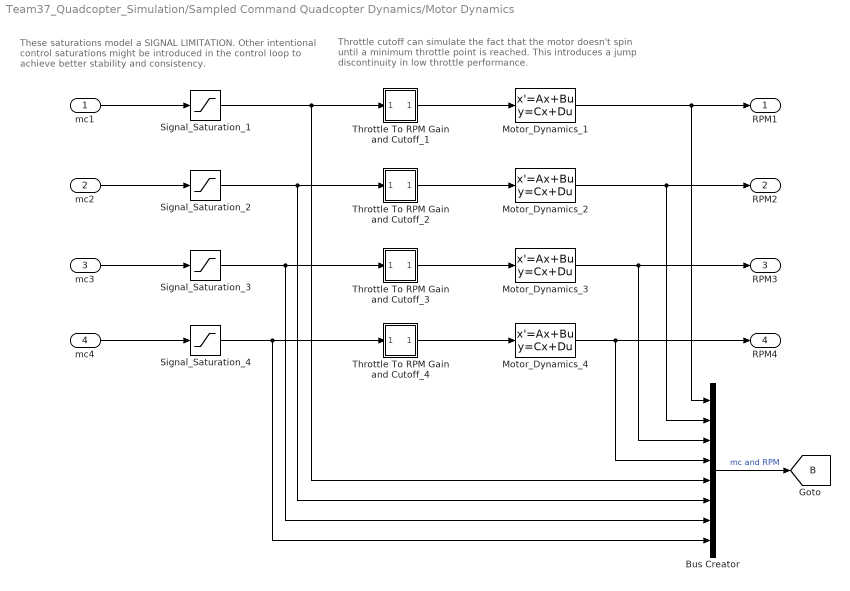
== system Team37_Quadcopter_Simulation/Sampled Command Quadcopter Dynamics/Motor Dynamics ==
  note: Throttle cutoff can simulate the fact that the motor doesn't
      | spin until a minimum throttle point is reached. This introduces
      | a jump discontinuity in low throttle performance.
  note: These saturations model a SIGNAL LIMITATION.
      | Other intentional control saturations might be introduced in the
      | control loop to achieve better stability and consistency.
  mc1 : Inport
  mc2 : Inport  Port=2
  mc3 : Inport  Port=3
  mc4 : Inport  Port=4
  Bus Creator : BusCreator  Inputs=8
  Motor_Dynamics_1 : StateSpace  A=-1/quadModel.T  C=1/quadModel.T  D=0  InitialCondition=IC.w1*quadModel.T
  Motor_Dynamics_2 : StateSpace  A=-1/quadModel.T  C=1/quadModel.T  D=0  InitialCondition=IC.w2*quadModel.T
  Motor_Dynamics_3 : StateSpace  A=-1/quadModel.T  C=1/quadModel.T  D=0  InitialCondition=IC.w3*quadModel.T
  Motor_Dynamics_4 : StateSpace  A=-1/quadModel.T  C=1/quadModel.T  D=0  InitialCondition=IC.w4*quadModel.T
  Signal_Saturation_{1..4} (4 alike) : Saturate  UpperLimit=100  LowerLimit=0
  Throttle To RPM Gain and Cutoff_1 : Subsystem
  Throttle To RPM Gain and Cutoff_2 : Subsystem
  Throttle To RPM Gain and Cutoff_3 : Subsystem
  Throttle To RPM Gain and Cutoff_4 : Subsystem
  RPM1 : Outport
  RPM2 : Outport  Port=2
  RPM3 : Outport  Port=3
  RPM4 : Outport  Port=4
  tag scope: B=global
  wires:
  mc1/1 -> Signal_Saturation_1/1
  mc4/1 -> Signal_Saturation_4/1
  mc2/1 -> Signal_Saturation_2/1
  mc3/1 -> Signal_Saturation_3/1
  Signal_Saturation_1/1 -> Bus Creator/5, Throttle To RPM Gain and Cutoff_1/1(In5)
  Signal_Saturation_2/1 -> Bus Creator/6, Throttle To RPM Gain and Cutoff_2/1(In5)
  Signal_Saturation_3/1 -> Bus Creator/7, Throttle To RPM Gain and Cutoff_3/1(In5)
  Signal_Saturation_4/1 -> Bus Creator/8, Throttle To RPM Gain and Cutoff_4/1(In5)
  Throttle To RPM Gain and Cutoff_1/1(Out5) -> Motor_Dynamics_1/1
  Throttle To RPM Gain and Cutoff_2/1(Out5) -> Motor_Dynamics_2/1
  Throttle To RPM Gain and Cutoff_3/1(Out5) -> Motor_Dynamics_3/1
  Throttle To RPM Gain and Cutoff_4/1(Out5) -> Motor_Dynamics_4/1
  Motor_Dynamics_1/1 -> Bus Creator/1, RPM1/1
  Motor_Dynamics_2/1 -> Bus Creator/2, RPM2/1
  Motor_Dynamics_3/1 -> Bus Creator/3, RPM3/1
  Motor_Dynamics_4/1 -> Bus Creator/4, RPM4/1
  Bus Creator/1 -> [B]  "mc and RPM"

== system Team37_Quadcopter_Simulation/Attitude Controller/Altitude (Z) Control/Derivative IC fixer ==
  FilterStart : Inport
  Normal Output : Inport  Port=2
  Constant : Constant
  IC : InitialCondition  Value=0
  Switch : Switch  Criteria=u2 ~= 0
  Out1 : Outport
  wires:
  Switch/1 -> Out1/1
  FilterStart/1 -> Switch/3
  IC/1 -> Switch/2
  Constant/1 -> IC/1
  Normal Output/1 -> Switch/1

== system Team37_Quadcopter_Simulation/On-board State Estimation/Mix Bus Output/Debug Scopes For Comparing Actual Versus Estimated Outputs This illustrates some of the effects from filtering ==
  note: Estimated are yellow, magenta are real
  note: Compare Outputs
  Estimated : Inport
  Actual : Inport  Port=2
  Bus Selector : BusSelector  OutputSignals=P,Q,R,Phi,The,Psi
  Bus Selector3 : BusSelector  OutputSignals=P,Q,R,Phi,The,Psi
  Mux{,1..5} (6 alike) : Mux  Inputs=2
  Scope : Scope  NumInputPorts=3
  Scope1 : Scope  NumInputPorts=3
  wires:
  Actual/1 -> Bus Selector3/1
  Mux5/1 -> Scope1/3
  Estimated/1 -> Bus Selector/1
  Bus Selector3/2 -> Mux4/2  "<Q>"
  Mux3/1 -> Scope1/1
  Mux4/1 -> Scope1/2
  Bus Selector/1 -> Mux3/1  "<P>"
  Bus Selector3/1 -> Mux3/2  "<P>"
  Bus Selector3/5 -> Mux1/2  "<The>"
  Bus Selector/3 -> Mux5/1  "<R>"
  Bus Selector/6 -> Mux2/1  "<Psi>"
  Bus Selector/2 -> Mux4/1  "<Q>"
  Mux2/1 -> Scope/3
  Bus Selector/5 -> Mux1/1  "<The>"
  Bus Selector/4 -> Mux/1  "<Phi>"
  Bus Selector3/3 -> Mux5/2  "<R>"
  Bus Selector3/6 -> Mux2/2  "<Psi>"
  Mux/1 -> Scope/1
  Mux1/1 -> Scope/2
  Bus Selector3/4 -> Mux/2  "<Phi>"

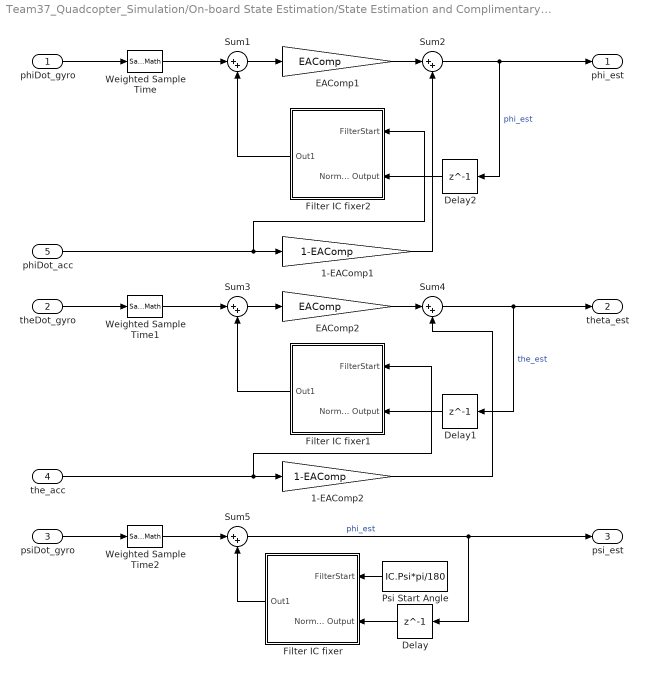
== system Team37_Quadcopter_Simulation/On-board State Estimation/State Estimation and Complimentary Mixing/Complimentary Filter ==
  phiDot_gyro : Inport
  theDot_gyro : Inport  Port=2
  psiDot_gyro : Inport  Port=3
  the_acc : Inport  Port=4
  phiDot_acc : Inport  Port=5
  1-EAComp1 : Gain  Gain=1-EAComp
  1-EAComp2 : Gain  Gain=1-EAComp
  Delay : Delay  DelayLength=1  InitialCondition=0
  Delay1 : Delay  DelayLength=1  InitialCondition=0
  Delay2 : Delay  DelayLength=1  InitialCondition=0
  EAComp1 : Gain  Gain=EAComp
  EAComp2 : Gain  Gain=EAComp
  Filter IC fixer : Subsystem
  Filter IC fixer1 : Subsystem
  Filter IC fixer2 : Subsystem
  Psi Start Angle : Constant  Value=IC.Psi*pi/180
  Sum{1..5} (5 alike) : Sum  Inputs=|++
  Weighted Sample Time : SampleTimeMath  TsampMathOp=*
  Weighted Sample Time1 : SampleTimeMath  TsampMathOp=*
  Weighted Sample Time2 : SampleTimeMath  TsampMathOp=*
  phi_est : Outport
  theta_est : Outport  Port=2
  psi_est : Outport  Port=3
  wires:
  Weighted Sample Time/1 -> Sum1/1
  Sum1/1 -> EAComp1/1
  Sum2/1 -> Delay2/1, phi_est/1  "phi_est"
  1-EAComp1/1 -> Sum2/2
  phiDot_gyro/1 -> Weighted Sample Time/1
  phiDot_acc/1 -> Filter IC fixer2/1(FilterStart), 1-EAComp1/1
  EAComp1/1 -> Sum2/1
  Weighted Sample Time1/1 -> Sum3/1
  Sum3/1 -> EAComp2/1
  Sum4/1 -> Delay1/1, theta_est/1  "the_est"
  1-EAComp2/1 -> Sum4/2
  theDot_gyro/1 -> Weighted Sample Time1/1
  the_acc/1 -> 1-EAComp2/1, Filter IC fixer1/1(FilterStart)
  EAComp2/1 -> Sum4/1
  psiDot_gyro/1 -> Weighted Sample Time2/1
  Weighted Sample Time2/1 -> Sum5/1
  Sum5/1 -> Delay/1, psi_est/1  "phi_est"
  Delay/1 -> Filter IC fixer/2(Normal Output)
  Filter IC fixer/1(Out1) -> Sum5/2
  Psi Start Angle/1 -> Filter IC fixer/1(FilterStart)
  Filter IC fixer1/1(Out1) -> Sum3/2
  Filter IC fixer2/1(Out1) -> Sum1/2
  Delay1/1 -> Filter IC fixer1/2(Normal Output)
  Delay2/1 -> Filter IC fixer2/2(Normal Output)

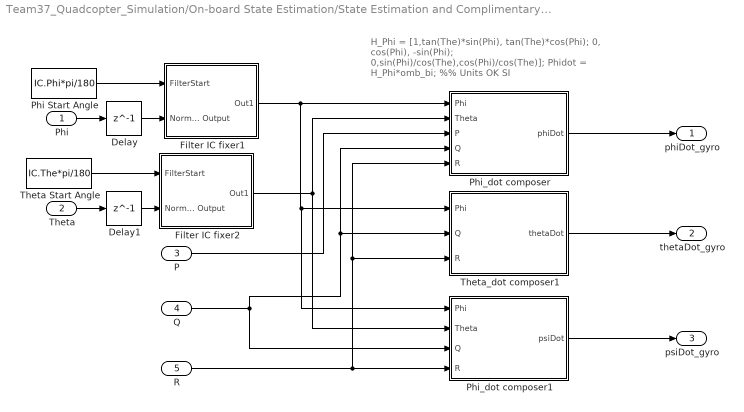
== system Team37_Quadcopter_Simulation/On-board State Estimation/State Estimation and Complimentary Mixing/Subsystem ==
  note: H_Phi = [1,tan(The)*sin(Phi), tan(The)*cos(Phi);
      |          0,         cos(Phi),         -sin(Phi);
      |          0,sin(Phi)/cos(The),cos(Phi)/cos(The)];
      | Phidot = H_Phi*omb_bi; %% Units OK SI
  Phi : Inport
  Theta : Inport  Port=2
  P : Inport  Port=3
  Q : Inport  Port=4
  R : Inport  Port=5
  Delay : Delay  DelayLength=1  InitialCondition=0
  Delay1 : Delay  DelayLength=1  InitialCondition=0
  Filter IC fixer1 : Subsystem
  Filter IC fixer2 : Subsystem
  Phi Start Angle : Constant  Value=IC.Phi*pi/180
  Phi_dot composer : Subsystem
  Phi_dot composer1 : Subsystem
  Theta Start Angle : Constant  Value=IC.The*pi/180
  Theta_dot composer1 : Subsystem
  phiDot_gyro : Outport
  thetaDot_gyro : Outport  Port=2
  psiDot_gyro : Outport  Port=3
  wires:
  P/1 -> Phi_dot composer/3(P)
  Q/1 -> Phi_dot composer1/3(Q), Theta_dot composer1/2(Q), Phi_dot composer/4(Q)
  Phi_dot composer/1(phiDot) -> phiDot_gyro/1
  Theta_dot composer1/1(thetaDot) -> thetaDot_gyro/1
  R/1 -> Theta_dot composer1/3(R), Phi_dot composer/5(R), Phi_dot composer1/4(R)
  Phi_dot composer1/1(psiDot) -> psiDot_gyro/1
  Filter IC fixer1/1(Out1) -> Phi_dot composer1/1(Phi), Theta_dot composer1/1(Phi), Phi_dot composer/1(Phi)
  Delay/1 -> Filter IC fixer1/2(Normal Output)
  Phi/1 -> Delay/1
  Phi Start Angle/1 -> Filter IC fixer1/1(FilterStart)
  Theta/1 -> Delay1/1
  Filter IC fixer2/1(Out1) -> Phi_dot composer/2(Theta), Phi_dot composer1/2(Theta)
  Delay1/1 -> Filter IC fixer2/2(Normal Output)
  Theta Start Angle/1 -> Filter IC fixer2/1(FilterStart)
